simulink model "sim5"  (R2022b)
settings: Solver=VariableStepAuto  StartTime=0.0  StopTime=czas_symulacji  RelTol=1e-3
values from neighbouring files (symbols this model uses):
  dqg = 0.1*qgN    (= 1000)    [Lab5.m]    (also in Lab5_wspolne_wykresy.m)
  dTzew = 1    [Lab5.m]    (also in Lab5_wspolne_wykresy.m)
  L11 = M2    [Lab5.m]    (also in Lab5_wspolne_wykresy.m)
  L12 = [kcw*Cvp kcp*kcwp+kcw*kcwp+kcw*kcp]    [Lab5.m]    (also in Lab5_wspolne_wykresy.m)
  L21 = kcwp    (= 69.7674418605)    [Lab5.m]    (also in Lab5_wspolne_wykresy.m)
  L22 = [kcp*Cvw kcwp*kcw+kcw*kcp+kcwp*kcp]    [Lab5.m]    (also in Lab5_wspolne_wykresy.m)
  M = [Cvw*Cvp Cvw*kcwp+Cvw*kcp+Cvp*kcw+Cvp*kcwp kcw*kcwp+kcw*kcp+kcwp*kcp]    [Lab5.m]    (also in Lab5_wspolne_wykresy.m)
  Tp0 = ((kcp*Tzew0)*(kcw+kcwp)+kcwp*(qg0+kcw*Tzew0))/(kcwp*kcw+kcp*kcw+kcp*kcwp)    [Lab5.m]    (also in Lab5_wspolne_wykresy.m)
  Twew0 = (qg0+kcw*Tzew0+kcwp*Tp0)/(kcw+kcwp)    [Lab5.m]    (also in Lab5_wspolne_wykresy.m)
settings Model: Creator=franc  LastModifiedBy=Dawkin
settings DataIOCC: ReturnWorkspaceOutputs=off

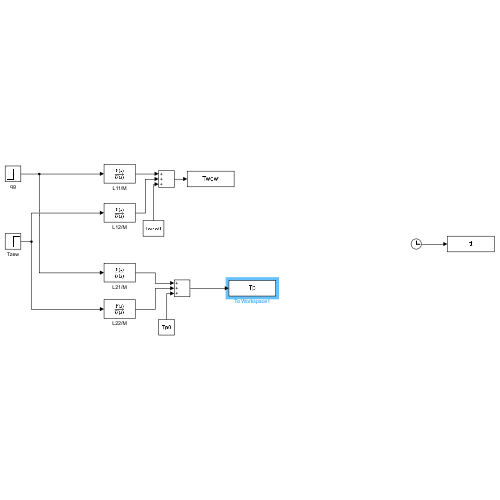
[thumbnail: Simulink's stored preview of the top-level diagram]
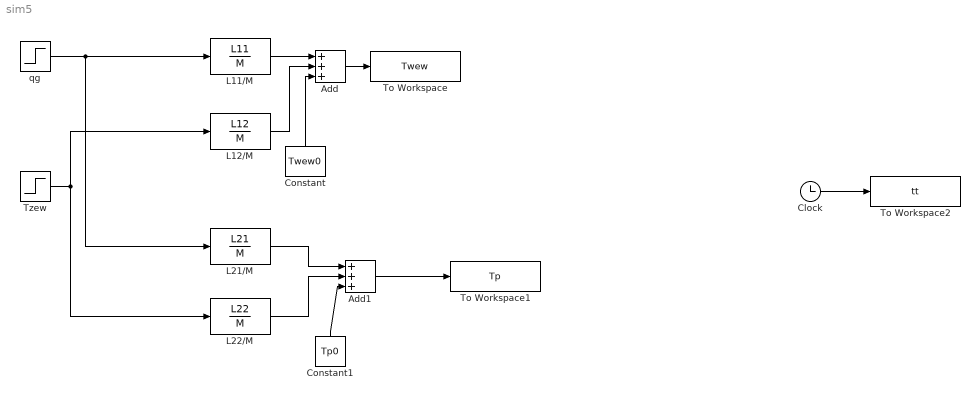
== system sim5 ==
  Add : Sum  Inputs=+++
  Add1 : Sum  Inputs=+++
  Clock : Clock
  Constant : Constant  Value=Twew0
  Constant1 : Constant  Value=Tp0
  L11/M : TransferFcn  Numerator=L11  Denominator=M
  L12/M : TransferFcn  Numerator=L12  Denominator=M
  L21/M : TransferFcn  Numerator=L21  Denominator=M
  L22/M : TransferFcn  Numerator=L22  Denominator=M
  To Workspace : ToWorkspace  VariableName=Twew  SampleTime=-1
  To Workspace1 : ToWorkspace  VariableName=Tp  SampleTime=-1
  To Workspace2 : ToWorkspace  VariableName=tt  SaveFormat=Timeseries  SampleTime=-1
  Tzew : Step  After=dTzew  SampleTime=0
  qg : Step  After=dqg  SampleTime=0
  wires:
  qg/1 -> L21/M/1, L11/M/1
  L11/M/1 -> Add/1
  Tzew/1 -> L22/M/1, L12/M/1
  L12/M/1 -> Add/2
  Add/1 -> To Workspace/1
  L21/M/1 -> Add1/1
  L22/M/1 -> Add1/2
  Add1/1 -> To Workspace1/1
  Clock/1 -> To Workspace2/1
  Constant/1 -> Add/3
  Constant1/1 -> Add1/3
